simulink model "phxex_sim_sorter"  (R2026a)
settings: Solver=FixedStepDiscrete  StopTime=60  FixedStep=0.005
values from neighbouring files (symbols this model uses):
  Trap = phx.Body("Type", "kinematic", "Position", [16.00 0 zc(16.00)], "EulerAngles", [0 deg2rad(20) 0], "Shape", {"Box", "Size", [5.5 9 0.4], "Color", [0.20 0.80 0.40]}, "Friction", [0.1 0 0], "Name", "Trap")    [model_sorter.m]
libraries: PhxLibrary x2, simulink x2
settings Model: Creator=lzhan  LastModifiedBy=lzhan
settings DebuggingCC: UnderspecifiedInitializationDetection=Classic
settings SimscapeCC: SimscapeNominalValues="[{\"value\":\"1\",\"unit\":\"A\"},{\"value\":\"1\",\"unit\":\"bar\"},{\"value\":\"1\",\"unit\":\"cm^2\"},{\"value\":\"1\",\"unit\":\"cm^3/s\"},{\"value\":\"1\",\"unit\":\"kJ/kg\"},{\"value\":\"1\",\"unit\":\"kW\"},{\"value\":\"1\",\"unit\":\"l\"},{\"value\":\"1\",\"unit\":\"N\"},{\"value\":\"1\",\"unit\":\"N*m\"},{\"value\":\"1\",\"unit\":\"V\"}]"  SimscapeLogType=none  SimscapeLogDataHistory=5000.0

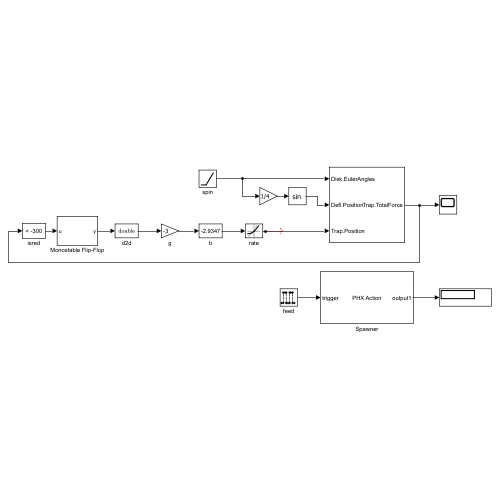
[thumbnail: Simulink's stored preview of the top-level diagram]
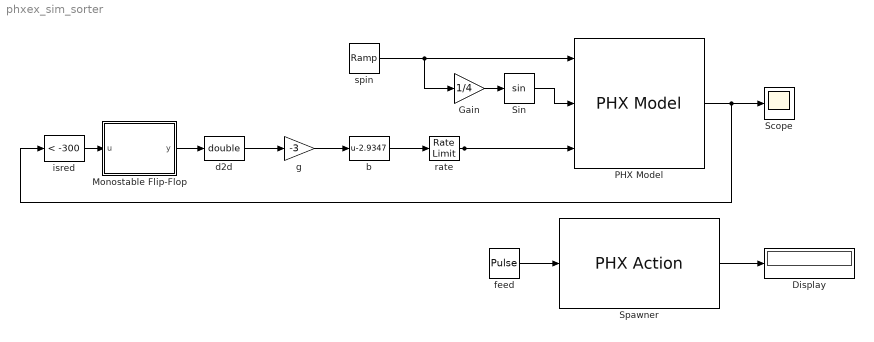
== system phxex_sim_sorter ==
  Display : Display
  Gain : Gain  Gain=1/4
  Monostable Flip-Flop : Subsystem
  PHX Model : PhxLibrary/PHX Model  ModelSource=saved_sorter.mat  InputRefs=|  OutputRefs=Trap.TotalForce(3)  ShowViewer=on  RenderEach=on  CameraPosition=[12 -24 45]  CameraTarget=[12 0 -3]  SimulationStep=0.01  SimpleIcon=off  Substeps=1  CameraResolution=[0 0]
      | Disk.EulerAngles(3)
      | Defl.Position(2)
      | Trap.Position(3)
      settings: SourceProductName=PHX Toolbox
  Scope : Scope
      settings: ActiveDisplayYMinimum=-1307.748981608896  ActiveDisplayYMaximum=145.30544240098843
  Sin : Trigonometry
  Spawner : PhxLibrary/PHX Action  Code=|  NumInputs=0  OutputSizes={1}  MainBlock=22
      | if ~isfield(state,'parts'); state.parts = struct('b',{},'red',{}); state.n = 0; end
      | state.n = state.n + 1;
      | isRed = mod(state.n,2)==1;
      | c = [0.3 0.5 0.9]; if isRed; c = [0.9 0.3 0.3]; end
      | b = phx.Body(ax, "Position", [0 5.0 2.5], "Shape", {"Box","Size",[1.2 1.2 1.2],"Density",1+isRed*2,"Color",c}, "Friction",[0.9 0.05 0]);
      | sim.addObjects(b);
      | output1=state.n;
      settings: SourceProductName=PHX Toolbox
  b : Bias  Bias=-2.9347  SaturateOnIntegerOverflow=off
  d2d : DataTypeConversion  OutDataTypeStr=double  SaturateOnIntegerOverflow=off  RndMeth=Floor
  feed : DiscretePulseGenerator  Period=60  PulseWidth=30  SampleTime=0.05
  g : Gain  Gain=-3
  isred : simulink/Logic and Bit Operations/Compare To Constant  relop=<  const=-300  OutDataTypeStr=boolean
  rate : RateLimiter  RisingSlewLimit=10  FallingSlewLimit=-20  SampleTimeMode=inherited
  spin : simulink/Sources/Ramp  slope=0.7  start=0  InitialOutput=0
  wires:
  d2d/1 -> g/1
  Spawner/1 -> Display/1
  feed/1 -> Spawner/1
  b/1 -> rate/1
  g/1 -> b/1
  rate/1 -> PHX Model/3
  spin/1 -> Gain/1, PHX Model/1
  PHX Model/1 -> isred/1, Scope/1
  isred/1 -> Monostable Flip-Flop/1(u)
  Monostable Flip-Flop/1(y) -> d2d/1
  Sin/1 -> PHX Model/2
  Gain/1 -> Sin/1

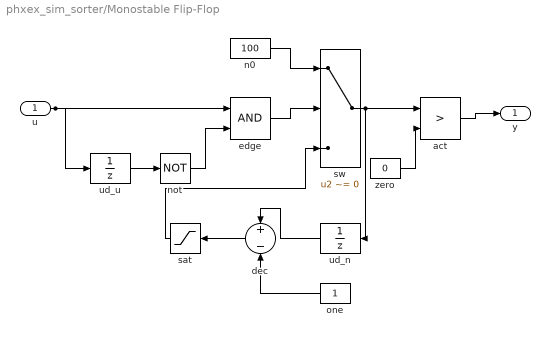
== system phxex_sim_sorter/Monostable Flip-Flop ==
  u : Inport
  act : RelationalOperator  Operator=>
  dec : Sum  Inputs=+-
  edge : Logic
  n0 : Constant  Value=100
  not : Logic  Operator=NOT
  one : Constant
  sat : Saturate  UpperLimit=inf  LowerLimit=0
  sw : Switch  Criteria=u2 ~= 0
  ud_n : UnitDelay  SampleTime=0.01
  ud_u : UnitDelay  SampleTime=0.01
  zero : Constant  Value=0
  y : Outport
  wires:
  u/1 -> edge/1, ud_u/1
  ud_u/1 -> not/1
  not/1 -> edge/2
  edge/1 -> sw/2
  n0/1 -> sw/1
  sw/1 -> act/1, ud_n/1
  ud_n/1 -> dec/1
  one/1 -> dec/2
  dec/1 -> sat/1
  sat/1 -> sw/3
  zero/1 -> act/2
  act/1 -> y/1
